simulink model "triggered"  (R2014a)
settings: Solver=ode3  StartTime=0.0  StopTime=Inf  FixedStep=0.2  RelTol=1e-3
undefined symbols (not defined in the file): DiscIntNeverNeededParam
libraries: simulink x1
settings Model: Creator=eruffaldi  LastModifiedBy=eruffaldi

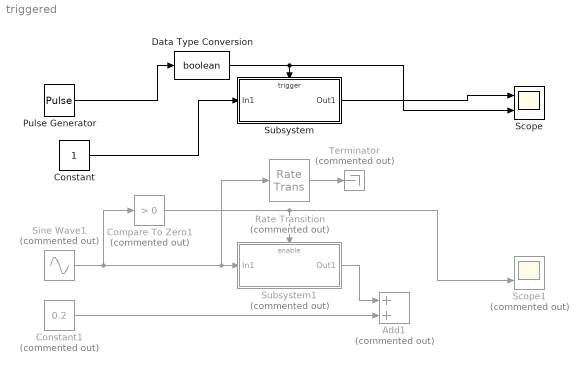
== system triggered ==
  Add1 : Sum  Commented=on
  Compare To Zero1 : simulink/Logic and Bit Operations/Compare To Zero  Commented=on  relop=>  OutDataTypeStr=boolean
  Constant : Constant
  Constant1 : Constant  Commented=on  Value=0.2
  Data Type Conversion : DataTypeConversion  OutDataTypeStr=boolean  SaturateOnIntegerOverflow=on  RndMeth=Zero
  Pulse Generator : DiscretePulseGenerator  PulseType=Time based  Period=10  PulseWidth=5
  Rate Transition : RateTransition  Commented=on
  Scope : Scope  NumInputPorts=2
      settings: YMin=-5~-5  YMax=5~5
  Scope1 : Scope  Commented=on  NumInputPorts=2
      settings: YMin=-5~-5  YMax=5~5
  Sine Wave1 : Sin  Commented=on  SampleTime=0.2
  Subsystem : Subsystem
  Subsystem1 : Subsystem  Commented=on
  Terminator : Terminator  Commented=on
  wires:
  Pulse Generator/1 -> Data Type Conversion/1
  Subsystem/1(Out1) -> Scope/1
  Sine Wave1/1 -> Rate Transition/1, Subsystem1/1(In1), Compare To Zero1/1
  Compare To Zero1/1 -> Scope1/2, Subsystem1/Enable
  Constant1/1 -> Add1/2
  Subsystem1/1(Out1) -> Add1/1
  Rate Transition/1 -> Terminator/1
  Data Type Conversion/1 -> Subsystem/Trigger, Scope/2
  Constant/1 -> Subsystem/1(In1)

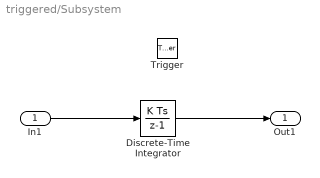
== system triggered/Subsystem ==
  In1 : Inport
  Trigger : TriggerPort  TriggerType=either  PortDimensions=1
  Discrete-Time Integrator : DiscreteIntegrator  SampleTime=-1  ICPrevOutput=DiscIntNeverNeededParam  ICPrevScaledInput=DiscIntNeverNeededParam
  Out1 : Outport
  wires:
  In1/1 -> Discrete-Time Integrator/1
  Discrete-Time Integrator/1 -> Out1/1

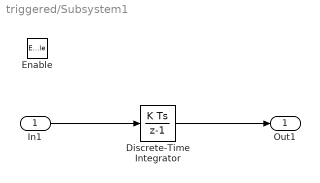
== system triggered/Subsystem1 ==
  In1 : Inport
  Enable : EnablePort
  Discrete-Time Integrator : DiscreteIntegrator  SampleTime=-1  ICPrevOutput=DiscIntNeverNeededParam  ICPrevScaledInput=DiscIntNeverNeededParam
  Out1 : Outport
  wires:
  In1/1 -> Discrete-Time Integrator/1
  Discrete-Time Integrator/1 -> Out1/1
